simulink model "ES102A_PolarityCfg"
settings: Solver=ode45  StartTime=0.0  StopTime=10.0  RelTol=1e-3
undefined symbols (not defined in the file or in its folder): sigbuilder_block
libraries: simulink x29
(part 2 of 4)

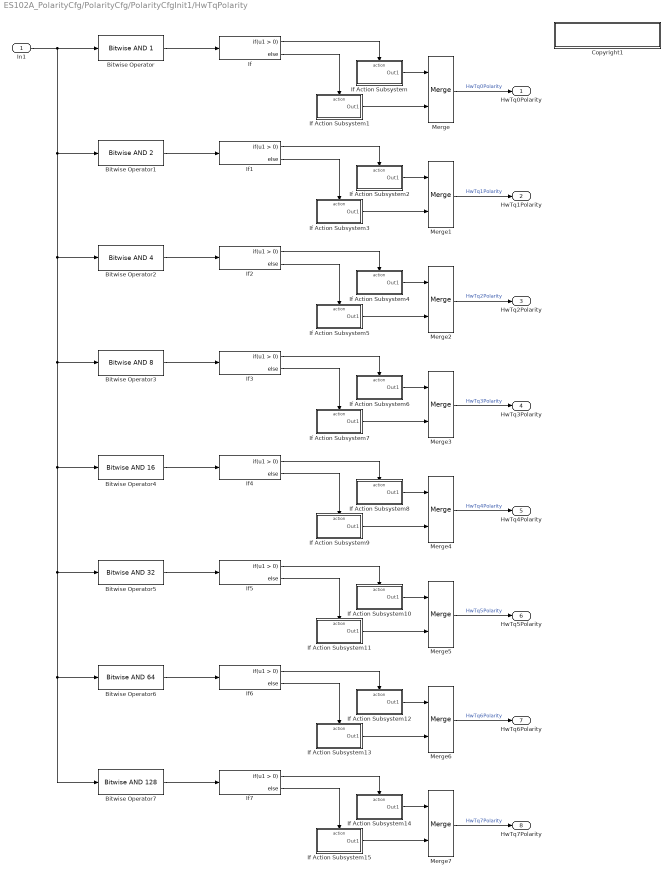
== system ES102A_PolarityCfg/PolarityCfg/PolarityCfgInit1/HwTqPolarity ==
  In1 : Inport
  Bitwise Operator : simulink/Logic and Bit Operations/Bitwise Operator  logicop=AND  UseBitMask=on  BitMask=1  BitMaskRealWorld=Stored Integer
  Bitwise Operator1 : simulink/Logic and Bit Operations/Bitwise Operator  logicop=AND  UseBitMask=on  BitMask=2  BitMaskRealWorld=Stored Integer
  Bitwise Operator2 : simulink/Logic and Bit Operations/Bitwise Operator  logicop=AND  UseBitMask=on  BitMask=4  BitMaskRealWorld=Stored Integer
  Bitwise Operator3 : simulink/Logic and Bit Operations/Bitwise Operator  logicop=AND  UseBitMask=on  BitMask=8  BitMaskRealWorld=Stored Integer
  Bitwise Operator4 : simulink/Logic and Bit Operations/Bitwise Operator  logicop=AND  UseBitMask=on  BitMask=16  BitMaskRealWorld=Stored Integer
  Bitwise Operator5 : simulink/Logic and Bit Operations/Bitwise Operator  logicop=AND  UseBitMask=on  BitMask=32  BitMaskRealWorld=Stored Integer
  Bitwise Operator6 : simulink/Logic and Bit Operations/Bitwise Operator  logicop=AND  UseBitMask=on  BitMask=64  BitMaskRealWorld=Stored Integer
  Bitwise Operator7 : simulink/Logic and Bit Operations/Bitwise Operator  logicop=AND  UseBitMask=on  BitMask=128  BitMaskRealWorld=Stored Integer
  Copyright1 : Subsystem  Description=|  mask(Copyright Information){none=on}
      | Copyright info block.                                               
      |                                                                     
      | Place copyright information at the top of every subsystem in design.
      mask prompts: none "No parameters"
      mask help: Place copyright information at the top of every subsystem in design.
      mask Display:
      | NxtrConf = 'Nexteer Confidential';
      | 
      | sys = bdroot; %handle for the current model ("system")
      | first = get_param(sys,'Created');
      | if(isempty(first))
      |     first = datestr(now,'yyyy');
      | else
      |     first = first(end-3:end);  %year is last four digits
      | end
      | 
      | last = get_param(sys,'LastModifiedDate');
      | if isempty(last)
      |     last = datestr(now,'yyyy');
      | else
      |     last = last(end-3:end);
      | end
      | 
      | if strcmp(first,last)
      |     fprintf('%s\nCopyright  %s Nexteer',NxtrConf,first);
      | else
      |     fprintf('%s\n%s%s-%s Nexteer',NxtrConf,char(169),first,last);
      | end
  If{,1..7} (8 alike) : If
  If Action Subsystem : Subsystem  RequirementInfo={'linktype_rmi_doors' '0000c464 (/ESG Group/FDD Module Requirements/EA4 Specific/ES102A_PolarityCfg_Draft)' '#ES102A_80' 'true' 'REQ: ES102A_80' '' } %GIDa_63d7a222_87e2_4426_b4d4_26a598cfd3d3  TreatAsAtomicUnit=on
  If Action Subsystem1 : Subsystem  RequirementInfo={'linktype_rmi_doors' '0000c464 (/ESG Group/FDD Module Requirements/EA4 Specific/ES102A_PolarityCfg_Draft)' '#ES102A_120' 'true' 'REQ: ES102A_120' '' } %GIDa_21104850_c1b3_421f_933d_f5e3d512e7eb  TreatAsAtomicUnit=on
  If Action Subsystem10 : Subsystem  RequirementInfo={'linktype_rmi_doors' '0000c464 (/ESG Group/FDD Module Requirements/EA4 Specific/ES102A_PolarityCfg_Draft)' '#ES102A_80' 'true' 'REQ: ES102A_80' '' } %GIDa_d3816962_365d_4dbe_9085_fe030921f526  TreatAsAtomicUnit=on
  If Action Subsystem11 : Subsystem  RequirementInfo={'linktype_rmi_doors' '0000c464 (/ESG Group/FDD Module Requirements/EA4 Specific/ES102A_PolarityCfg_Draft)' '#ES102A_120' 'true' 'REQ: ES102A_120' '' } %GIDa_f8f3beb7_25e0_4963_84bd_d008adb7cee4  TreatAsAtomicUnit=on
  If Action Subsystem12 : Subsystem  RequirementInfo={'linktype_rmi_doors' '0000c464 (/ESG Group/FDD Module Requirements/EA4 Specific/ES102A_PolarityCfg_Draft)' '#ES102A_80' 'true' 'REQ: ES102A_80' '' } %GIDa_2ee8a515_44ef_45e2_9975_0d23b295e5d1  TreatAsAtomicUnit=on
  If Action Subsystem13 : Subsystem  RequirementInfo={'linktype_rmi_doors' '0000c464 (/ESG Group/FDD Module Requirements/EA4 Specific/ES102A_PolarityCfg_Draft)' '#ES102A_120' 'true' 'REQ: ES102A_120' '' } %GIDa_ba2a0d96_0e4a_4325_88ca_f247a322979d  TreatAsAtomicUnit=on
  If Action Subsystem14 : Subsystem  RequirementInfo={'linktype_rmi_doors' '0000c464 (/ESG Group/FDD Module Requirements/EA4 Specific/ES102A_PolarityCfg_Draft)' '#ES102A_80' 'true' 'REQ: ES102A_80' '' } %GIDa_1f54eaba_6bb6_4127_a31e_ea55fd3abc1f  TreatAsAtomicUnit=on
  If Action Subsystem15 : Subsystem  RequirementInfo={'linktype_rmi_doors' '0000c464 (/ESG Group/FDD Module Requirements/EA4 Specific/ES102A_PolarityCfg_Draft)' '#ES102A_120' 'true' 'REQ: ES102A_120' '' } %GIDa_c83b58a0_3a0a_4eb5_80bd_66a98f93a285  TreatAsAtomicUnit=on
  If Action Subsystem2 : Subsystem  RequirementInfo={'linktype_rmi_doors' '0000c464 (/ESG Group/FDD Module Requirements/EA4 Specific/ES102A_PolarityCfg_Draft)' '#ES102A_80' 'true' 'REQ: ES102A_80' '' } %GIDa_5262a54c_aaf5_4732_b7ff_1f31c1412e9d  TreatAsAtomicUnit=on
  If Action Subsystem3 : Subsystem  RequirementInfo={'linktype_rmi_doors' '0000c464 (/ESG Group/FDD Module Requirements/EA4 Specific/ES102A_PolarityCfg_Draft)' '#ES102A_120' 'true' 'REQ: ES102A_120' '' } %GIDa_935cd820_58dd_45b1_8f3d_8d9b6ade2195  TreatAsAtomicUnit=on
  If Action Subsystem4 : Subsystem  RequirementInfo={'linktype_rmi_doors' '0000c464 (/ESG Group/FDD Module Requirements/EA4 Specific/ES102A_PolarityCfg_Draft)' '#ES102A_80' 'true' 'REQ: ES102A_80' '' } %GIDa_75b8dd12_95a3_44d6_8e99_0d6e0e3fdd6f  TreatAsAtomicUnit=on
  If Action Subsystem5 : Subsystem  RequirementInfo={'linktype_rmi_doors' '0000c464 (/ESG Group/FDD Module Requirements/EA4 Specific/ES102A_PolarityCfg_Draft)' '#ES102A_120' 'true' 'REQ: ES102A_120' '' } %GIDa_379eacf7_c184_4183_bde5_d58bfea1b961  TreatAsAtomicUnit=on
  If Action Subsystem6 : Subsystem  RequirementInfo={'linktype_rmi_doors' '0000c464 (/ESG Group/FDD Module Requirements/EA4 Specific/ES102A_PolarityCfg_Draft)' '#ES102A_80' 'true' 'REQ: ES102A_80' '' } %GIDa_93f31a74_0cd9_423c_8377_1edcd093e5d6  TreatAsAtomicUnit=on
  If Action Subsystem7 : Subsystem  RequirementInfo={'linktype_rmi_doors' '0000c464 (/ESG Group/FDD Module Requirements/EA4 Specific/ES102A_PolarityCfg_Draft)' '#ES102A_120' 'true' 'REQ: ES102A_120' '' } %GIDa_60e8f548_0e62_4727_b735_42e2eee2da9c  TreatAsAtomicUnit=on
  If Action Subsystem8 : Subsystem  RequirementInfo={'linktype_rmi_doors' '0000c464 (/ESG Group/FDD Module Requirements/EA4 Specific/ES102A_PolarityCfg_Draft)' '#ES102A_80' 'true' 'REQ: ES102A_80' '' } %GIDa_48fc852b_25d9_48ef_8317_b5544d331087  TreatAsAtomicUnit=on
  If Action Subsystem9 : Subsystem  RequirementInfo={'linktype_rmi_doors' '0000c464 (/ESG Group/FDD Module Requirements/EA4 Specific/ES102A_PolarityCfg_Draft)' '#ES102A_120' 'true' 'REQ: ES102A_120' '' } %GIDa_afefc9ee_dd4f_448b_8cdc_7ccd5a68edf1  TreatAsAtomicUnit=on
  Merge : Merge  RequirementInfo={'linktype_rmi_doors' '0000c464 (/ESG Group/FDD Module Requirements/EA4 Specific/ES102A_PolarityCfg_Draft)' '#ES102A_51' 'true' 'REQ: ES102A_51' '' } %GIDa_f47d43ed_cc5a_434e_8d3d_13b3ba273cfe
  Merge1 : Merge  RequirementInfo={'linktype_rmi_doors' '0000c464 (/ESG Group/FDD Module Requirements/EA4 Specific/ES102A_PolarityCfg_Draft)' '#ES102A_96' 'true' 'REQ: ES102A_96' '' } %GIDa_e39f7e38_3c59_4e11_80bf_3cfa32d59145
  Merge2 : Merge  RequirementInfo={'linktype_rmi_doors' '0000c464 (/ESG Group/FDD Module Requirements/EA4 Specific/ES102A_PolarityCfg_Draft)' '#ES102A_97' 'true' 'REQ: ES102A_97' '' } %GIDa_656ea733_9417_4392_8103_592feb91c3e2
  Merge3 : Merge  RequirementInfo={'linktype_rmi_doors' '0000c464 (/ESG Group/FDD Module Requirements/EA4 Specific/ES102A_PolarityCfg_Draft)' '#ES102A_98' 'true' 'REQ: ES102A_98' '' } %GIDa_67ab4764_dfdf_4d10_ad00_44d5b6543dad
  Merge4 : Merge  RequirementInfo={'linktype_rmi_doors' '0000c464 (/ESG Group/FDD Module Requirements/EA4 Specific/ES102A_PolarityCfg_Draft)' '#ES102A_99' 'true' 'REQ: ES102A_99' '' } %GIDa_f01d10c9_6713_4a58_8677_254d13779cb8
  Merge5 : Merge  RequirementInfo={'linktype_rmi_doors' '0000c464 (/ESG Group/FDD Module Requirements/EA4 Specific/ES102A_PolarityCfg_Draft)' '#ES102A_100' 'true' 'REQ: ES102A_100' '' } %GIDa_b89c6608_65de_4443_9860_b993d639af9c
  Merge6 : Merge  RequirementInfo={'linktype_rmi_doors' '0000c464 (/ESG Group/FDD Module Requirements/EA4 Specific/ES102A_PolarityCfg_Draft)' '#ES102A_101' 'true' 'REQ: ES102A_101' '' } %GIDa_62c0d5ff_61a3_4196_82ea_7ef23e77f0bd
  Merge7 : Merge  RequirementInfo={'linktype_rmi_doors' '0000c464 (/ESG Group/FDD Module Requirements/EA4 Specific/ES102A_PolarityCfg_Draft)' '#ES102A_102' 'true' 'REQ: ES102A_102' '' } %GIDa_3c3479f6_5363_44fc_9164_2b7c4fbc1053
  HwTq0Polarity : Outport  RequirementInfo={'doors' '00006113' '48' 'false' 'DOORS Surrogate Item' '' ; 'linktype_rmi_doors' '0000c464 (/ESG Group/FDD Module Requirements/EA4 Specific/ES102A_PolarityCfg_Draft)' '#ES102A_51' 'true' 'REQ: ES102A_51' '' } %GIDa_c470d9f1_1471_4152_8210_a7d10d57422b
  HwTq1Polarity : Outport  RequirementInfo={'doors' '00006113' '49' 'false' 'DOORS Surrogate Item' '' ; 'linktype_rmi_doors' '0000c464 (/ESG Group/FDD Module Requirements/EA4 Specific/ES102A_PolarityCfg_Draft)' '#ES102A_96' 'true' 'REQ: ES102A_96' '' } %GIDa_ed40a89e_763c_4172_ae71_4f4717fd1c6c  Port=2
  HwTq2Polarity : Outport  RequirementInfo={'doors' '00006113' '50' 'false' 'DOORS Surrogate Item' '' ; 'linktype_rmi_doors' '0000c464 (/ESG Group/FDD Module Requirements/EA4 Specific/ES102A_PolarityCfg_Draft)' '#ES102A_97' 'true' 'REQ: ES102A_97' '' } %GIDa_7620c17f_03f2_4abd_85dc_4468565938e3  Port=3
  HwTq3Polarity : Outport  RequirementInfo={'doors' '00006113' '51' 'false' 'DOORS Surrogate Item' '' ; 'linktype_rmi_doors' '0000c464 (/ESG Group/FDD Module Requirements/EA4 Specific/ES102A_PolarityCfg_Draft)' '#ES102A_98' 'true' 'REQ: ES102A_98' '' } %GIDa_eb5c760f_4214_4ac8_9392_ece161eb896a  Port=4
  HwTq4Polarity : Outport  RequirementInfo={'doors' '00006113' '52' 'false' 'DOORS Surrogate Item' '' ; 'linktype_rmi_doors' '0000c464 (/ESG Group/FDD Module Requirements/EA4 Specific/ES102A_PolarityCfg_Draft)' '#ES102A_99' 'true' 'REQ: ES102A_99' '' } %GIDa_111b98a5_5481_44e8_b0fd_d626e710aa2c  Port=5
  HwTq5Polarity : Outport  RequirementInfo={'doors' '00006113' '53' 'false' 'DOORS Surrogate Item' '' ; 'linktype_rmi_doors' '0000c464 (/ESG Group/FDD Module Requirements/EA4 Specific/ES102A_PolarityCfg_Draft)' '#ES102A_100' 'true' 'REQ: ES102A_100' '' } %GIDa_95f59e0f_aa02_4d07_be0c_357d651a5e8c  Port=6
  HwTq6Polarity : Outport  RequirementInfo={'doors' '00006113' '54' 'false' 'DOORS Surrogate Item' '' ; 'linktype_rmi_doors' '0000c464 (/ESG Group/FDD Module Requirements/EA4 Specific/ES102A_PolarityCfg_Draft)' '#ES102A_101' 'true' 'REQ: ES102A_101' '' } %GIDa_e6057f56_db9b_40f9_aef9_186face4720b  Port=7
  HwTq7Polarity : Outport  RequirementInfo={'doors' '00006113' '55' 'false' 'DOORS Surrogate Item' '' ; 'linktype_rmi_doors' '0000c464 (/ESG Group/FDD Module Requirements/EA4 Specific/ES102A_PolarityCfg_Draft)' '#ES102A_102' 'true' 'REQ: ES102A_102' '' } %GIDa_37c293f9_76a2_48d9_8980_8af8f7443fdf  Port=8
  wires:
  Bitwise Operator/1 -> If/1
  If/1 -> If Action Subsystem/Action
  If/2 -> If Action Subsystem1/Action
  If Action Subsystem/1(Out1) -> Merge/1
  If Action Subsystem1/1(Out1) -> Merge/2
  Merge/1 -> HwTq0Polarity/1  "HwTq0Polarity"
  Bitwise Operator1/1 -> If1/1
  If1/1 -> If Action Subsystem2/Action
  If1/2 -> If Action Subsystem3/Action
  If Action Subsystem2/1(Out1) -> Merge1/1
  If Action Subsystem3/1(Out1) -> Merge1/2
  Merge1/1 -> HwTq1Polarity/1  "HwTq1Polarity"
  Bitwise Operator2/1 -> If2/1
  If2/1 -> If Action Subsystem4/Action
  If2/2 -> If Action Subsystem5/Action
  If Action Subsystem4/1(Out1) -> Merge2/1
  If Action Subsystem5/1(Out1) -> Merge2/2
  Merge2/1 -> HwTq2Polarity/1  "HwTq2Polarity"
  Bitwise Operator3/1 -> If3/1
  If3/1 -> If Action Subsystem6/Action
  If3/2 -> If Action Subsystem7/Action
  If Action Subsystem6/1(Out1) -> Merge3/1
  If Action Subsystem7/1(Out1) -> Merge3/2
  Merge3/1 -> HwTq3Polarity/1  "HwTq3Polarity"
  Bitwise Operator4/1 -> If4/1
  If4/1 -> If Action Subsystem8/Action
  If4/2 -> If Action Subsystem9/Action
  If Action Subsystem8/1(Out1) -> Merge4/1
  If Action Subsystem9/1(Out1) -> Merge4/2
  Merge4/1 -> HwTq4Polarity/1  "HwTq4Polarity"
  Bitwise Operator5/1 -> If5/1
  If5/1 -> If Action Subsystem10/Action
  If5/2 -> If Action Subsystem11/Action
  If Action Subsystem10/1(Out1) -> Merge5/1
  If Action Subsystem11/1(Out1) -> Merge5/2
  Merge5/1 -> HwTq5Polarity/1  "HwTq5Polarity"
  In1/1 -> Bitwise Operator2/1, Bitwise Operator7/1, Bitwise Operator6/1, Bitwise Operator5/1, Bitwise Operator4/1, Bitwise Operator3/1, Bitwise Operator1/1, Bitwise Operator/1
  Bitwise Operator6/1 -> If6/1
  If6/1 -> If Action Subsystem12/Action
  If6/2 -> If Action Subsystem13/Action
  If Action Subsystem12/1(Out1) -> Merge6/1
  If Action Subsystem13/1(Out1) -> Merge6/2
  Merge6/1 -> HwTq6Polarity/1  "HwTq6Polarity"
  Bitwise Operator7/1 -> If7/1
  If7/1 -> If Action Subsystem14/Action
  If7/2 -> If Action Subsystem15/Action
  If Action Subsystem14/1(Out1) -> Merge7/1
  If Action Subsystem15/1(Out1) -> Merge7/2
  Merge7/1 -> HwTq7Polarity/1  "HwTq7Polarity"

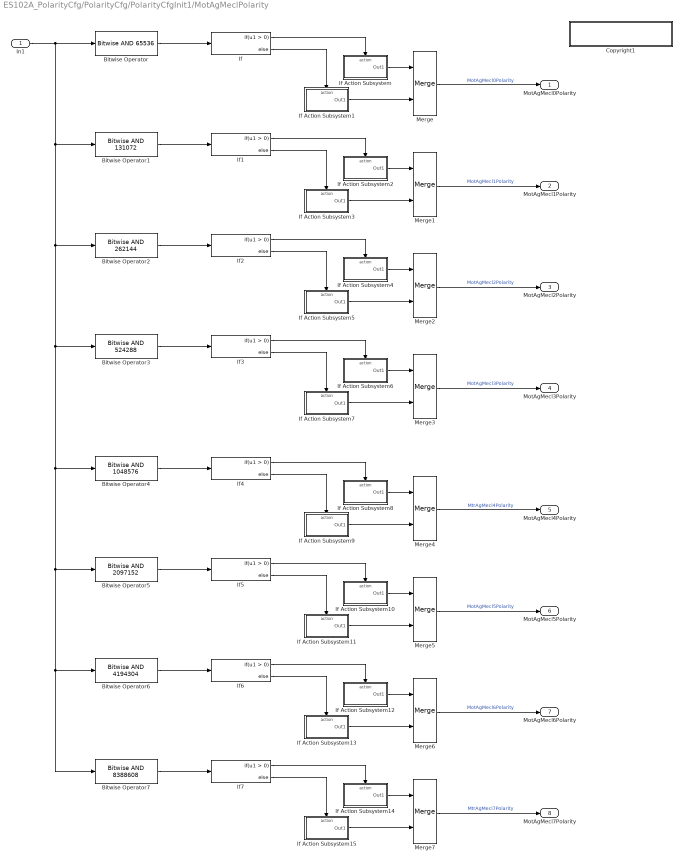
== system ES102A_PolarityCfg/PolarityCfg/PolarityCfgInit1/MotAgMeclPolarity ==
  In1 : Inport
  Bitwise Operator : simulink/Logic and Bit Operations/Bitwise Operator  logicop=AND  UseBitMask=on  BitMask=65536  BitMaskRealWorld=Stored Integer
  Bitwise Operator1 : simulink/Logic and Bit Operations/Bitwise Operator  logicop=AND  UseBitMask=on  BitMask=131072  BitMaskRealWorld=Stored Integer
  Bitwise Operator2 : simulink/Logic and Bit Operations/Bitwise Operator  logicop=AND  UseBitMask=on  BitMask=262144  BitMaskRealWorld=Stored Integer
  Bitwise Operator3 : simulink/Logic and Bit Operations/Bitwise Operator  logicop=AND  UseBitMask=on  BitMask=524288  BitMaskRealWorld=Stored Integer
  Bitwise Operator4 : simulink/Logic and Bit Operations/Bitwise Operator  logicop=AND  UseBitMask=on  BitMask=1048576  BitMaskRealWorld=Stored Integer
  Bitwise Operator5 : simulink/Logic and Bit Operations/Bitwise Operator  logicop=AND  UseBitMask=on  BitMask=2097152  BitMaskRealWorld=Stored Integer
  Bitwise Operator6 : simulink/Logic and Bit Operations/Bitwise Operator  logicop=AND  UseBitMask=on  BitMask=4194304  BitMaskRealWorld=Stored Integer
  Bitwise Operator7 : simulink/Logic and Bit Operations/Bitwise Operator  logicop=AND  UseBitMask=on  BitMask=8388608  BitMaskRealWorld=Stored Integer
  Copyright1 : Subsystem  Description=|  mask(Copyright Information){none=on}
      | Copyright info block.                                               
      |                                                                     
      | Place copyright information at the top of every subsystem in design.
      mask prompts: none "No parameters"
      mask help: Place copyright information at the top of every subsystem in design.
      mask Display:
      | NxtrConf = 'Nexteer Confidential';
      | 
      | sys = bdroot; %handle for the current model ("system")
      | first = get_param(sys,'Created');
      | if(isempty(first))
      |     first = datestr(now,'yyyy');
      | else
      |     first = first(end-3:end);  %year is last four digits
      | end
      | 
      | last = get_param(sys,'LastModifiedDate');
      | if isempty(last)
      |     last = datestr(now,'yyyy');
      | else
      |     last = last(end-3:end);
      | end
      | 
      | if strcmp(first,last)
      |     fprintf('%s\nCopyright  %s Nexteer',NxtrConf,first);
      | else
      |     fprintf('%s\n%s%s-%s Nexteer',NxtrConf,char(169),first,last);
      | end
  If{,1..7} (8 alike) : If
  If Action Subsystem : Subsystem  RequirementInfo={'linktype_rmi_doors' '0000c464 (/ESG Group/FDD Module Requirements/EA4 Specific/ES102A_PolarityCfg_Draft)' '#ES102A_80' 'true' 'REQ: ES102A_80' '' } %GIDa_c5946f2f_0b9f_4812_9390_249c5458628f  TreatAsAtomicUnit=on
  If Action Subsystem1 : Subsystem  RequirementInfo={'linktype_rmi_doors' '0000c464 (/ESG Group/FDD Module Requirements/EA4 Specific/ES102A_PolarityCfg_Draft)' '#ES102A_120' 'true' 'REQ: ES102A_120' '' } %GIDa_17235a92_0b57_4ead_b18c_bc699b71e168  TreatAsAtomicUnit=on
  If Action Subsystem10 : Subsystem  RequirementInfo={'linktype_rmi_doors' '0000c464 (/ESG Group/FDD Module Requirements/EA4 Specific/ES102A_PolarityCfg_Draft)' '#ES102A_80' 'true' 'REQ: ES102A_80' '' } %GIDa_cabfc731_1079_4863_87d4_a2a1f3eed74c  TreatAsAtomicUnit=on
  If Action Subsystem11 : Subsystem  RequirementInfo={'linktype_rmi_doors' '0000c464 (/ESG Group/FDD Module Requirements/EA4 Specific/ES102A_PolarityCfg_Draft)' '#ES102A_120' 'true' 'REQ: ES102A_120' '' } %GIDa_de40052c_f86a_4ed6_a4cf_70244dc4a80a  TreatAsAtomicUnit=on
  If Action Subsystem12 : Subsystem  RequirementInfo={'linktype_rmi_doors' '0000c464 (/ESG Group/FDD Module Requirements/EA4 Specific/ES102A_PolarityCfg_Draft)' '#ES102A_80' 'true' 'REQ: ES102A_80' '' } %GIDa_6ed3d26d_6828_4944_90c2_e0466ba8cbfc  TreatAsAtomicUnit=on
  If Action Subsystem13 : Subsystem  RequirementInfo={'linktype_rmi_doors' '0000c464 (/ESG Group/FDD Module Requirements/EA4 Specific/ES102A_PolarityCfg_Draft)' '#ES102A_120' 'true' 'REQ: ES102A_120' '' } %GIDa_520226fe_c2b8_4250_b652_b1e7aaf239e5  TreatAsAtomicUnit=on
  If Action Subsystem14 : Subsystem  RequirementInfo={'linktype_rmi_doors' '0000c464 (/ESG Group/FDD Module Requirements/EA4 Specific/ES102A_PolarityCfg_Draft)' '#ES102A_80' 'true' 'REQ: ES102A_80' '' } %GIDa_9f63c0d2_98df_422d_9e76_08480bd61c35  TreatAsAtomicUnit=on
  If Action Subsystem15 : Subsystem  RequirementInfo={'linktype_rmi_doors' '0000c464 (/ESG Group/FDD Module Requirements/EA4 Specific/ES102A_PolarityCfg_Draft)' '#ES102A_120' 'true' 'REQ: ES102A_120' '' } %GIDa_c6055289_5356_4833_a678_20f7ef84d772  TreatAsAtomicUnit=on
  If Action Subsystem2 : Subsystem  RequirementInfo={'linktype_rmi_doors' '0000c464 (/ESG Group/FDD Module Requirements/EA4 Specific/ES102A_PolarityCfg_Draft)' '#ES102A_80' 'true' 'REQ: ES102A_80' '' } %GIDa_0192eca6_12f5_480b_91b0_5cfcc8faccb1  TreatAsAtomicUnit=on
  If Action Subsystem3 : Subsystem  RequirementInfo={'linktype_rmi_doors' '0000c464 (/ESG Group/FDD Module Requirements/EA4 Specific/ES102A_PolarityCfg_Draft)' '#ES102A_120' 'true' 'REQ: ES102A_120' '' } %GIDa_d6d5d98a_008b_4639_ba1e_e67d332e29db  TreatAsAtomicUnit=on
  If Action Subsystem4 : Subsystem  RequirementInfo={'linktype_rmi_doors' '0000c464 (/ESG Group/FDD Module Requirements/EA4 Specific/ES102A_PolarityCfg_Draft)' '#ES102A_80' 'true' 'REQ: ES102A_80' '' } %GIDa_3d5fefbf_36ef_4545_87b2_e45a305df674  TreatAsAtomicUnit=on
  If Action Subsystem5 : Subsystem  RequirementInfo={'linktype_rmi_doors' '0000c464 (/ESG Group/FDD Module Requirements/EA4 Specific/ES102A_PolarityCfg_Draft)' '#ES102A_120' 'true' 'REQ: ES102A_120' '' } %GIDa_361beeaf_56ac_433f_8adf_074565dfac65  TreatAsAtomicUnit=on
  If Action Subsystem6 : Subsystem  RequirementInfo={'linktype_rmi_doors' '0000c464 (/ESG Group/FDD Module Requirements/EA4 Specific/ES102A_PolarityCfg_Draft)' '#ES102A_80' 'true' 'REQ: ES102A_80' '' } %GIDa_8efca514_65fe_4817_8fbf_cf5f41ffb619  TreatAsAtomicUnit=on
  If Action Subsystem7 : Subsystem  RequirementInfo={'linktype_rmi_doors' '0000c464 (/ESG Group/FDD Module Requirements/EA4 Specific/ES102A_PolarityCfg_Draft)' '#ES102A_120' 'true' 'REQ: ES102A_120' '' } %GIDa_073176ef_7645_42c7_a94e_900cce625b51  TreatAsAtomicUnit=on
  If Action Subsystem8 : Subsystem  RequirementInfo={'linktype_rmi_doors' '0000c464 (/ESG Group/FDD Module Requirements/EA4 Specific/ES102A_PolarityCfg_Draft)' '#ES102A_80' 'true' 'REQ: ES102A_80' '' } %GIDa_59e259d9_ce1e_4f89_b54a_b64fcb6e78a8  TreatAsAtomicUnit=on
  If Action Subsystem9 : Subsystem  RequirementInfo={'linktype_rmi_doors' '0000c464 (/ESG Group/FDD Module Requirements/EA4 Specific/ES102A_PolarityCfg_Draft)' '#ES102A_120' 'true' 'REQ: ES102A_120' '' } %GIDa_52fcd065_e02d_4289_8673_fa8d1da08e21  TreatAsAtomicUnit=on
  Merge : Merge  RequirementInfo={'linktype_rmi_doors' '0000c464 (/ESG Group/FDD Module Requirements/EA4 Specific/ES102A_PolarityCfg_Draft)' '#ES102A_111' 'true' 'REQ: ES102A_111' '' } %GIDa_1cb9118c_0659_4e90_9a33_0e30e3279ea9
  Merge1 : Merge  RequirementInfo={'linktype_rmi_doors' '0000c464 (/ESG Group/FDD Module Requirements/EA4 Specific/ES102A_PolarityCfg_Draft)' '#ES102A_112' 'true' 'REQ: ES102A_112' '' } %GIDa_01804cea_1b6c_4f32_b834_efb460ab85bd
  Merge2 : Merge  RequirementInfo={'linktype_rmi_doors' '0000c464 (/ESG Group/FDD Module Requirements/EA4 Specific/ES102A_PolarityCfg_Draft)' '#ES102A_113' 'true' 'REQ: ES102A_113' '' } %GIDa_206dd265_0520_4812_b6ee_41059434edda
  Merge3 : Merge  RequirementInfo={'linktype_rmi_doors' '0000c464 (/ESG Group/FDD Module Requirements/EA4 Specific/ES102A_PolarityCfg_Draft)' '#ES102A_114' 'true' 'REQ: ES102A_114' '' } %GIDa_3fafbf9e_b20c_4e77_94f2_328bf7bc39b3
  Merge4 : Merge  RequirementInfo={'linktype_rmi_doors' '0000c464 (/ESG Group/FDD Module Requirements/EA4 Specific/ES102A_PolarityCfg_Draft)' '#ES102A_115' 'true' 'REQ: ES102A_115' '' } %GIDa_7ec066e2_acbd_43a3_b4bc_fc416caebe36
  Merge5 : Merge  RequirementInfo={'linktype_rmi_doors' '0000c464 (/ESG Group/FDD Module Requirements/EA4 Specific/ES102A_PolarityCfg_Draft)' '#ES102A_116' 'true' 'REQ: ES102A_116' '' } %GIDa_e8cb3a86_3d61_44d4_805c_75ed0ab79821
  Merge6 : Merge  RequirementInfo={'linktype_rmi_doors' '0000c464 (/ESG Group/FDD Module Requirements/EA4 Specific/ES102A_PolarityCfg_Draft)' '#ES102A_117' 'true' 'REQ: ES102A_117' '' } %GIDa_625fcab5_94af_4caf_8215_0ddb1120ff87
  Merge7 : Merge  RequirementInfo={'linktype_rmi_doors' '0000c464 (/ESG Group/FDD Module Requirements/EA4 Specific/ES102A_PolarityCfg_Draft)' '#ES102A_118' 'true' 'REQ: ES102A_118' '' } %GIDa_92dfed0d_b9ba_4979_87bf_08f80fe7be37
  MotAgMecl0Polarity : Outport  RequirementInfo={'doors' '00006113' '73' 'false' 'DOORS Surrogate Item' '' ; 'linktype_rmi_doors' '0000c464 (/ESG Group/FDD Module Requirements/EA4 Specific/ES102A_PolarityCfg_Draft)' '#ES102A_111' 'true' 'REQ: ES102A_111' '' } %GIDa_95216d83_d457_4bf2_af30_873833492705
  MotAgMecl1Polarity : Outport  RequirementInfo={'doors' '00006113' '74' 'false' 'DOORS Surrogate Item' '' ; 'linktype_rmi_doors' '0000c464 (/ESG Group/FDD Module Requirements/EA4 Specific/ES102A_PolarityCfg_Draft)' '#ES102A_112' 'true' 'REQ: ES102A_112' '' } %GIDa_ff0e6218_2686_4598_b6b7_fa5f98e64f97  Port=2
  MotAgMecl2Polarity : Outport  RequirementInfo={'doors' '00006113' '75' 'false' 'DOORS Surrogate Item' '' ; 'linktype_rmi_doors' '0000c464 (/ESG Group/FDD Module Requirements/EA4 Specific/ES102A_PolarityCfg_Draft)' '#ES102A_113' 'true' 'REQ: ES102A_113' '' } %GIDa_7394a991_4a99_40ff_9081_355143f46542  Port=3
  MotAgMecl3Polarity : Outport  RequirementInfo={'doors' '00006113' '76' 'false' 'DOORS Surrogate Item' '' ; 'linktype_rmi_doors' '0000c464 (/ESG Group/FDD Module Requirements/EA4 Specific/ES102A_PolarityCfg_Draft)' '#ES102A_114' 'true' 'REQ: ES102A_114' '' } %GIDa_da4aeb3a_9c72_4710_9d7a_5d798e9d90a7  Port=4
  MotAgMecl4Polarity : Outport  RequirementInfo={'doors' '00006113' '77' 'false' 'DOORS Surrogate Item' '' ; 'linktype_rmi_doors' '0000c464 (/ESG Group/FDD Module Requirements/EA4 Specific/ES102A_PolarityCfg_Draft)' '#ES102A_115' 'true' 'REQ: ES102A_115' '' } %GIDa_88a06b38_1492_417e_b5eb_cfb04e1c5553  Port=5
  MotAgMecl5Polarity : Outport  RequirementInfo={'doors' '00006113' '78' 'false' 'DOORS Surrogate Item' '' ; 'linktype_rmi_doors' '0000c464 (/ESG Group/FDD Module Requirements/EA4 Specific/ES102A_PolarityCfg_Draft)' '#ES102A_116' 'true' 'REQ: ES102A_116' '' } %GIDa_e6f50b59_6521_4921_86d4_3e49b0dfffd0  Port=6
  MotAgMecl6Polarity : Outport  RequirementInfo={'doors' '00006113' '79' 'false' 'DOORS Surrogate Item' '' ; 'linktype_rmi_doors' '0000c464 (/ESG Group/FDD Module Requirements/EA4 Specific/ES102A_PolarityCfg_Draft)' '#ES102A_117' 'true' 'REQ: ES102A_117' '' } %GIDa_afa3a81b_308b_4dd4_a88d_b812527054d6  Port=7
  MotAgMecl7Polarity : Outport  RequirementInfo={'doors' '00006113' '80' 'false' 'DOORS Surrogate Item' '' ; 'linktype_rmi_doors' '0000c464 (/ESG Group/FDD Module Requirements/EA4 Specific/ES102A_PolarityCfg_Draft)' '#ES102A_118' 'true' 'REQ: ES102A_118' '' } %GIDa_a990ee8c_3420_4843_8508_80e3dc931edb  Port=8
  wires:
  Bitwise Operator/1 -> If/1
  If/1 -> If Action Subsystem/Action
  If/2 -> If Action Subsystem1/Action
  If Action Subsystem/1(Out1) -> Merge/1
  If Action Subsystem1/1(Out1) -> Merge/2
  Merge/1 -> MotAgMecl0Polarity/1  "MotAgMecl0Polarity"
  Bitwise Operator1/1 -> If1/1
  If1/1 -> If Action Subsystem2/Action
  If1/2 -> If Action Subsystem3/Action
  If Action Subsystem2/1(Out1) -> Merge1/1
  If Action Subsystem3/1(Out1) -> Merge1/2
  Merge1/1 -> MotAgMecl1Polarity/1  "MotAgMecl1Polarity"
  Bitwise Operator2/1 -> If2/1
  If2/1 -> If Action Subsystem4/Action
  If2/2 -> If Action Subsystem5/Action
  If Action Subsystem4/1(Out1) -> Merge2/1
  If Action Subsystem5/1(Out1) -> Merge2/2
  Merge2/1 -> MotAgMecl2Polarity/1  "MotAgMecl2Polarity"
  Bitwise Operator3/1 -> If3/1
  If3/1 -> If Action Subsystem6/Action
  If3/2 -> If Action Subsystem7/Action
  If Action Subsystem6/1(Out1) -> Merge3/1
  If Action Subsystem7/1(Out1) -> Merge3/2
  Merge3/1 -> MotAgMecl3Polarity/1  "MotAgMecl3Polarity"
  Bitwise Operator4/1 -> If4/1
  If4/1 -> If Action Subsystem8/Action
  If4/2 -> If Action Subsystem9/Action
  If Action Subsystem8/1(Out1) -> Merge4/1
  If Action Subsystem9/1(Out1) -> Merge4/2
  Merge4/1 -> MotAgMecl4Polarity/1  "MtrAgMecl4Polarity"
  Bitwise Operator5/1 -> If5/1
  If5/1 -> If Action Subsystem10/Action
  If5/2 -> If Action Subsystem11/Action
  If Action Subsystem10/1(Out1) -> Merge5/1
  If Action Subsystem11/1(Out1) -> Merge5/2
  Merge5/1 -> MotAgMecl5Polarity/1  "MotAgMecl5Polarity"
  In1/1 -> Bitwise Operator2/1, Bitwise Operator6/1, Bitwise Operator7/1, Bitwise Operator5/1, Bitwise Operator4/1, Bitwise Operator3/1, Bitwise Operator1/1, Bitwise Operator/1
  Bitwise Operator6/1 -> If6/1
  If6/1 -> If Action Subsystem12/Action
  If6/2 -> If Action Subsystem13/Action
  If Action Subsystem12/1(Out1) -> Merge6/1
  If Action Subsystem13/1(Out1) -> Merge6/2
  Merge6/1 -> MotAgMecl6Polarity/1  "MotAgMecl6Polarity"
  Bitwise Operator7/1 -> If7/1
  If7/1 -> If Action Subsystem14/Action
  If7/2 -> If Action Subsystem15/Action
  If Action Subsystem14/1(Out1) -> Merge7/1
  If Action Subsystem15/1(Out1) -> Merge7/2
  Merge7/1 -> MotAgMecl7Polarity/1  "MtrAgMecl7Polarity"

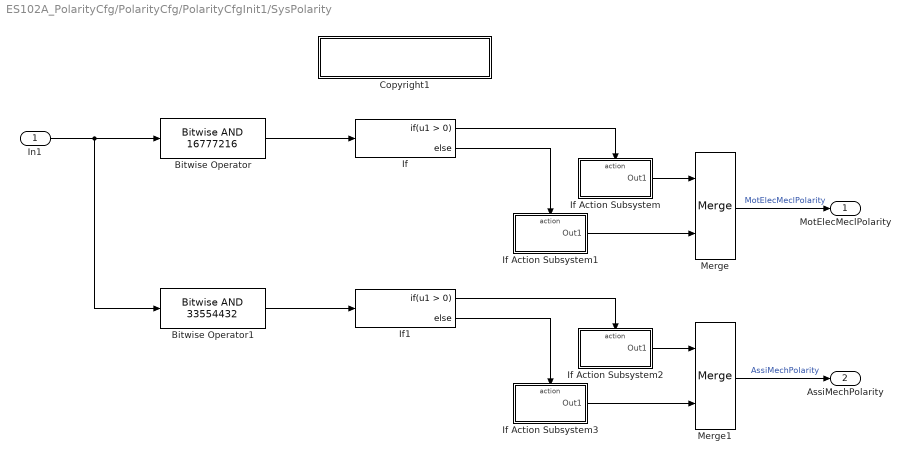
== system ES102A_PolarityCfg/PolarityCfg/PolarityCfgInit1/SysPolarity ==
  In1 : Inport
  Bitwise Operator : simulink/Logic and Bit Operations/Bitwise Operator  logicop=AND  UseBitMask=on  BitMask=16777216  BitMaskRealWorld=Stored Integer
  Bitwise Operator1 : simulink/Logic and Bit Operations/Bitwise Operator  logicop=AND  UseBitMask=on  BitMask=33554432  BitMaskRealWorld=Stored Integer
  Copyright1 : Subsystem  Description=|  mask(Copyright Information){none=on}
      | Copyright info block.                                               
      |                                                                     
      | Place copyright information at the top of every subsystem in design.
      mask prompts: none "No parameters"
      mask help: Place copyright information at the top of every subsystem in design.
      mask Display:
      | NxtrConf = 'Nexteer Confidential';
      | 
      | sys = bdroot; %handle for the current model ("system")
      | first = get_param(sys,'Created');
      | if(isempty(first))
      |     first = datestr(now,'yyyy');
      | else
      |     first = first(end-3:end);  %year is last four digits
      | end
      | 
      | last = get_param(sys,'LastModifiedDate');
      | if isempty(last)
      |     last = datestr(now,'yyyy');
      | else
      |     last = last(end-3:end);
      | end
      | 
      | if strcmp(first,last)
      |     fprintf('%s\nCopyright  %s Nexteer',NxtrConf,first);
      | else
      |     fprintf('%s\n%s%s-%s Nexteer',NxtrConf,char(169),first,last);
      | end
  If : If
  If Action Subsystem : Subsystem  RequirementInfo={'linktype_rmi_doors' '0000c464 (/ESG Group/FDD Module Requirements/EA4 Specific/ES102A_PolarityCfg_Draft)' '#ES102A_80' 'true' 'REQ: ES102A_80' '' } %GIDa_d9e8b945_10d8_4f4e_94d9_8ce26ac6b54b  TreatAsAtomicUnit=on
  If Action Subsystem1 : Subsystem  RequirementInfo={'linktype_rmi_doors' '0000c464 (/ESG Group/FDD Module Requirements/EA4 Specific/ES102A_PolarityCfg_Draft)' '#ES102A_120' 'true' 'REQ: ES102A_120' '' } %GIDa_bc435f67_2244_4529_9754_6b8f8d041ec6  TreatAsAtomicUnit=on
  If Action Subsystem2 : Subsystem  RequirementInfo={'linktype_rmi_doors' '0000c464 (/ESG Group/FDD Module Requirements/EA4 Specific/ES102A_PolarityCfg_Draft)' '#ES102A_80' 'true' 'REQ: ES102A_80' '' } %GIDa_fd742fd1_1f2e_4be3_9489_f2890f4a54eb  TreatAsAtomicUnit=on
  If Action Subsystem3 : Subsystem  RequirementInfo={'linktype_rmi_doors' '0000c464 (/ESG Group/FDD Module Requirements/EA4 Specific/ES102A_PolarityCfg_Draft)' '#ES102A_120' 'true' 'REQ: ES102A_120' '' } %GIDa_84388462_660c_472b_b9a9_b3c4ad928bf4  TreatAsAtomicUnit=on
  If1 : If
  Merge : Merge  RequirementInfo={'linktype_rmi_doors' '0000c464 (/ESG Group/FDD Module Requirements/EA4 Specific/ES102A_PolarityCfg_Draft)' '#ES102A_119' 'true' 'REQ: ES102A_119' '' } %GIDa_42684085_e280_43cc_93a1_7d0e1be79bcf
  Merge1 : Merge  RequirementInfo={'linktype_rmi_doors' '0000c464 (/ESG Group/FDD Module Requirements/EA4 Specific/ES102A_PolarityCfg_Draft)' '#ES102A_124' 'true' 'REQ: ES102A_124' '' } %GIDa_8f3b19c0_6ac2_44b0_9cf3_e074e9794d93
  MotElecMeclPolarity : Outport  RequirementInfo={'doors' '00006113' '98' 'false' 'DOORS Surrogate Item' '' ; 'linktype_rmi_doors' '0000c464 (/ESG Group/FDD Module Requirements/EA4 Specific/ES102A_PolarityCfg_Draft)' '#ES102A_119' 'true' 'REQ: ES102A_119' '' } %GIDa_fc271306_0e1e_4ad7_8e39_60fa997cde00
  AssiMechPolarity : Outport  RequirementInfo={'doors' '00006113' '99' 'false' 'DOORS Surrogate Item' '' ; 'linktype_rmi_doors' '0000c464 (/ESG Group/FDD Module Requirements/EA4 Specific/ES102A_PolarityCfg_Draft)' '#ES102A_124' 'true' 'REQ: ES102A_124' '' } %GIDa_29efb95d_12e9_44c1_aeec_7b34f9c231f1  Port=2
  wires:
  Bitwise Operator/1 -> If/1
  If/1 -> If Action Subsystem/Action
  If/2 -> If Action Subsystem1/Action
  If Action Subsystem/1(Out1) -> Merge/1
  If Action Subsystem1/1(Out1) -> Merge/2
  Merge/1 -> MotElecMeclPolarity/1  "MotElecMeclPolarity"
  Bitwise Operator1/1 -> If1/1
  If1/1 -> If Action Subsystem2/Action
  If1/2 -> If Action Subsystem3/Action
  If Action Subsystem2/1(Out1) -> Merge1/1
  If Action Subsystem3/1(Out1) -> Merge1/2
  Merge1/1 -> AssiMechPolarity/1  "AssiMechPolarity"
  In1/1 -> Bitwise Operator1/1, Bitwise Operator/1

== system ES102A_PolarityCfg/PolarityCfg/PolarityCfgRead/Copyright1 ==

== system ES102A_PolarityCfg/PolarityCfg/PolarityCfgWr/Copyright1 ==

== system ES102A_PolarityCfg/PolarityCfg/PolarityCfgWr/PolarityCfgSaved_SetRamBlockStatus ==
  note: This is the block representing the client call
  BlockChanged : Inport
  Terminator : Terminator
  wires:
  BlockChanged/1 -> Terminator/1

== system ES102A_PolarityCfg/PolarityCfg/PolarityCfgInit1/HwAgPolarity/Copyright1 ==

== system ES102A_PolarityCfg/PolarityCfg/PolarityCfgInit1/HwAgPolarity/If Action Subsystem ==
  Action Port : ActionPort  ActionType=then
  Constant : Constant
  Copyright1 : Subsystem  Description=|  mask(Copyright Information){none=on}
      | Copyright info block.                                               
      |                                                                     
      | Place copyright information at the top of every subsystem in design.
      mask prompts: none "No parameters"
      mask help: Place copyright information at the top of every subsystem in design.
      mask Display:
      | NxtrConf = 'Nexteer Confidential';
      | 
      | sys = bdroot; %handle for the current model ("system")
      | first = get_param(sys,'Created');
      | if(isempty(first))
      |     first = datestr(now,'yyyy');
      | else
      |     first = first(end-3:end);  %year is last four digits
      | end
      | 
      | last = get_param(sys,'LastModifiedDate');
      | if isempty(last)
      |     last = datestr(now,'yyyy');
      | else
      |     last = last(end-3:end);
      | end
      | 
      | if strcmp(first,last)
      |     fprintf('%s\nCopyright  %s Nexteer',NxtrConf,first);
      | else
      |     fprintf('%s\n%s%s-%s Nexteer',NxtrConf,char(169),first,last);
      | end
  Out1 : Outport  InitialOutput=1
  wires:
  Constant/1 -> Out1/1

== system ES102A_PolarityCfg/PolarityCfg/PolarityCfgInit1/HwAgPolarity/If Action Subsystem1 ==
  Action Port : ActionPort  ActionType=else
  Constant : Constant  Value=-1
  Copyright1 : Subsystem  Description=|  mask(Copyright Information){none=on}
      | Copyright info block.                                               
      |                                                                     
      | Place copyright information at the top of every subsystem in design.
      mask prompts: none "No parameters"
      mask help: Place copyright information at the top of every subsystem in design.
      mask Display:
      | NxtrConf = 'Nexteer Confidential';
      | 
      | sys = bdroot; %handle for the current model ("system")
      | first = get_param(sys,'Created');
      | if(isempty(first))
      |     first = datestr(now,'yyyy');
      | else
      |     first = first(end-3:end);  %year is last four digits
      | end
      | 
      | last = get_param(sys,'LastModifiedDate');
      | if isempty(last)
      |     last = datestr(now,'yyyy');
      | else
      |     last = last(end-3:end);
      | end
      | 
      | if strcmp(first,last)
      |     fprintf('%s\nCopyright  %s Nexteer',NxtrConf,first);
      | else
      |     fprintf('%s\n%s%s-%s Nexteer',NxtrConf,char(169),first,last);
      | end
  Out1 : Outport  InitialOutput=-1
  wires:
  Constant/1 -> Out1/1

== system ES102A_PolarityCfg/PolarityCfg/PolarityCfgInit1/HwAgPolarity/If Action Subsystem10 ==
  Action Port : ActionPort  ActionType=then
  Constant : Constant
  Copyright1 : Subsystem  Description=|  mask(Copyright Information){none=on}
      | Copyright info block.                                               
      |                                                                     
      | Place copyright information at the top of every subsystem in design.
      mask prompts: none "No parameters"
      mask help: Place copyright information at the top of every subsystem in design.
      mask Display:
      | NxtrConf = 'Nexteer Confidential';
      | 
      | sys = bdroot; %handle for the current model ("system")
      | first = get_param(sys,'Created');
      | if(isempty(first))
      |     first = datestr(now,'yyyy');
      | else
      |     first = first(end-3:end);  %year is last four digits
      | end
      | 
      | last = get_param(sys,'LastModifiedDate');
      | if isempty(last)
      |     last = datestr(now,'yyyy');
      | else
      |     last = last(end-3:end);
      | end
      | 
      | if strcmp(first,last)
      |     fprintf('%s\nCopyright  %s Nexteer',NxtrConf,first);
      | else
      |     fprintf('%s\n%s%s-%s Nexteer',NxtrConf,char(169),first,last);
      | end
  Out1 : Outport  InitialOutput=1
  wires:
  Constant/1 -> Out1/1

== system ES102A_PolarityCfg/PolarityCfg/PolarityCfgInit1/HwAgPolarity/If Action Subsystem11 ==
  Action Port : ActionPort  ActionType=else
  Constant : Constant  Value=-1
  Copyright1 : Subsystem  Description=|  mask(Copyright Information){none=on}
      | Copyright info block.                                               
      |                                                                     
      | Place copyright information at the top of every subsystem in design.
      mask prompts: none "No parameters"
      mask help: Place copyright information at the top of every subsystem in design.
      mask Display:
      | NxtrConf = 'Nexteer Confidential';
      | 
      | sys = bdroot; %handle for the current model ("system")
      | first = get_param(sys,'Created');
      | if(isempty(first))
      |     first = datestr(now,'yyyy');
      | else
      |     first = first(end-3:end);  %year is last four digits
      | end
      | 
      | last = get_param(sys,'LastModifiedDate');
      | if isempty(last)
      |     last = datestr(now,'yyyy');
      | else
      |     last = last(end-3:end);
      | end
      | 
      | if strcmp(first,last)
      |     fprintf('%s\nCopyright  %s Nexteer',NxtrConf,first);
      | else
      |     fprintf('%s\n%s%s-%s Nexteer',NxtrConf,char(169),first,last);
      | end
  Out1 : Outport  InitialOutput=-1
  wires:
  Constant/1 -> Out1/1

== system ES102A_PolarityCfg/PolarityCfg/PolarityCfgInit1/HwAgPolarity/If Action Subsystem12 ==
  Action Port : ActionPort  ActionType=then
  Constant : Constant
  Copyright1 : Subsystem  Description=|  mask(Copyright Information){none=on}
      | Copyright info block.                                               
      |                                                                     
      | Place copyright information at the top of every subsystem in design.
      mask prompts: none "No parameters"
      mask help: Place copyright information at the top of every subsystem in design.
      mask Display:
      | NxtrConf = 'Nexteer Confidential';
      | 
      | sys = bdroot; %handle for the current model ("system")
      | first = get_param(sys,'Created');
      | if(isempty(first))
      |     first = datestr(now,'yyyy');
      | else
      |     first = first(end-3:end);  %year is last four digits
      | end
      | 
      | last = get_param(sys,'LastModifiedDate');
      | if isempty(last)
      |     last = datestr(now,'yyyy');
      | else
      |     last = last(end-3:end);
      | end
      | 
      | if strcmp(first,last)
      |     fprintf('%s\nCopyright  %s Nexteer',NxtrConf,first);
      | else
      |     fprintf('%s\n%s%s-%s Nexteer',NxtrConf,char(169),first,last);
      | end
  Out1 : Outport  InitialOutput=1
  wires:
  Constant/1 -> Out1/1

== system ES102A_PolarityCfg/PolarityCfg/PolarityCfgInit1/HwAgPolarity/If Action Subsystem13 ==
  Action Port : ActionPort  ActionType=else
  Constant : Constant  Value=-1
  Copyright1 : Subsystem  Description=|  mask(Copyright Information){none=on}
      | Copyright info block.                                               
      |                                                                     
      | Place copyright information at the top of every subsystem in design.
      mask prompts: none "No parameters"
      mask help: Place copyright information at the top of every subsystem in design.
      mask Display:
      | NxtrConf = 'Nexteer Confidential';
      | 
      | sys = bdroot; %handle for the current model ("system")
      | first = get_param(sys,'Created');
      | if(isempty(first))
      |     first = datestr(now,'yyyy');
      | else
      |     first = first(end-3:end);  %year is last four digits
      | end
      | 
      | last = get_param(sys,'LastModifiedDate');
      | if isempty(last)
      |     last = datestr(now,'yyyy');
      | else
      |     last = last(end-3:end);
      | end
      | 
      | if strcmp(first,last)
      |     fprintf('%s\nCopyright  %s Nexteer',NxtrConf,first);
      | else
      |     fprintf('%s\n%s%s-%s Nexteer',NxtrConf,char(169),first,last);
      | end
  Out1 : Outport  InitialOutput=-1
  wires:
  Constant/1 -> Out1/1

== system ES102A_PolarityCfg/PolarityCfg/PolarityCfgInit1/HwAgPolarity/If Action Subsystem14 ==
  Action Port : ActionPort  ActionType=then
  Constant : Constant
  Copyright1 : Subsystem  Description=|  mask(Copyright Information){none=on}
      | Copyright info block.                                               
      |                                                                     
      | Place copyright information at the top of every subsystem in design.
      mask prompts: none "No parameters"
      mask help: Place copyright information at the top of every subsystem in design.
      mask Display:
      | NxtrConf = 'Nexteer Confidential';
      | 
      | sys = bdroot; %handle for the current model ("system")
      | first = get_param(sys,'Created');
      | if(isempty(first))
      |     first = datestr(now,'yyyy');
      | else
      |     first = first(end-3:end);  %year is last four digits
      | end
      | 
      | last = get_param(sys,'LastModifiedDate');
      | if isempty(last)
      |     last = datestr(now,'yyyy');
      | else
      |     last = last(end-3:end);
      | end
      | 
      | if strcmp(first,last)
      |     fprintf('%s\nCopyright  %s Nexteer',NxtrConf,first);
      | else
      |     fprintf('%s\n%s%s-%s Nexteer',NxtrConf,char(169),first,last);
      | end
  Out1 : Outport  InitialOutput=1
  wires:
  Constant/1 -> Out1/1

== system ES102A_PolarityCfg/PolarityCfg/PolarityCfgInit1/HwAgPolarity/If Action Subsystem15 ==
  Action Port : ActionPort  ActionType=else
  Constant : Constant  Value=-1
  Copyright1 : Subsystem  Description=|  mask(Copyright Information){none=on}
      | Copyright info block.                                               
      |                                                                     
      | Place copyright information at the top of every subsystem in design.
      mask prompts: none "No parameters"
      mask help: Place copyright information at the top of every subsystem in design.
      mask Display:
      | NxtrConf = 'Nexteer Confidential';
      | 
      | sys = bdroot; %handle for the current model ("system")
      | first = get_param(sys,'Created');
      | if(isempty(first))
      |     first = datestr(now,'yyyy');
      | else
      |     first = first(end-3:end);  %year is last four digits
      | end
      | 
      | last = get_param(sys,'LastModifiedDate');
      | if isempty(last)
      |     last = datestr(now,'yyyy');
      | else
      |     last = last(end-3:end);
      | end
      | 
      | if strcmp(first,last)
      |     fprintf('%s\nCopyright  %s Nexteer',NxtrConf,first);
      | else
      |     fprintf('%s\n%s%s-%s Nexteer',NxtrConf,char(169),first,last);
      | end
  Out1 : Outport  InitialOutput=-1
  wires:
  Constant/1 -> Out1/1

== system ES102A_PolarityCfg/PolarityCfg/PolarityCfgInit1/HwAgPolarity/If Action Subsystem2 ==
  Action Port : ActionPort  ActionType=then
  Constant : Constant
  Copyright1 : Subsystem  Description=|  mask(Copyright Information){none=on}
      | Copyright info block.                                               
      |                                                                     
      | Place copyright information at the top of every subsystem in design.
      mask prompts: none "No parameters"
      mask help: Place copyright information at the top of every subsystem in design.
      mask Display:
      | NxtrConf = 'Nexteer Confidential';
      | 
      | sys = bdroot; %handle for the current model ("system")
      | first = get_param(sys,'Created');
      | if(isempty(first))
      |     first = datestr(now,'yyyy');
      | else
      |     first = first(end-3:end);  %year is last four digits
      | end
      | 
      | last = get_param(sys,'LastModifiedDate');
      | if isempty(last)
      |     last = datestr(now,'yyyy');
      | else
      |     last = last(end-3:end);
      | end
      | 
      | if strcmp(first,last)
      |     fprintf('%s\nCopyright  %s Nexteer',NxtrConf,first);
      | else
      |     fprintf('%s\n%s%s-%s Nexteer',NxtrConf,char(169),first,last);
      | end
  Out1 : Outport  InitialOutput=1
  wires:
  Constant/1 -> Out1/1

== system ES102A_PolarityCfg/PolarityCfg/PolarityCfgInit1/HwAgPolarity/If Action Subsystem3 ==
  Action Port : ActionPort  ActionType=else
  Constant : Constant  Value=-1
  Copyright1 : Subsystem  Description=|  mask(Copyright Information){none=on}
      | Copyright info block.                                               
      |                                                                     
      | Place copyright information at the top of every subsystem in design.
      mask prompts: none "No parameters"
      mask help: Place copyright information at the top of every subsystem in design.
      mask Display:
      | NxtrConf = 'Nexteer Confidential';
      | 
      | sys = bdroot; %handle for the current model ("system")
      | first = get_param(sys,'Created');
      | if(isempty(first))
      |     first = datestr(now,'yyyy');
      | else
      |     first = first(end-3:end);  %year is last four digits
      | end
      | 
      | last = get_param(sys,'LastModifiedDate');
      | if isempty(last)
      |     last = datestr(now,'yyyy');
      | else
      |     last = last(end-3:end);
      | end
      | 
      | if strcmp(first,last)
      |     fprintf('%s\nCopyright  %s Nexteer',NxtrConf,first);
      | else
      |     fprintf('%s\n%s%s-%s Nexteer',NxtrConf,char(169),first,last);
      | end
  Out1 : Outport  InitialOutput=-1
  wires:
  Constant/1 -> Out1/1

== system ES102A_PolarityCfg/PolarityCfg/PolarityCfgInit1/HwAgPolarity/If Action Subsystem4 ==
  Action Port : ActionPort  ActionType=then
  Constant : Constant
  Copyright1 : Subsystem  Description=|  mask(Copyright Information){none=on}
      | Copyright info block.                                               
      |                                                                     
      | Place copyright information at the top of every subsystem in design.
      mask prompts: none "No parameters"
      mask help: Place copyright information at the top of every subsystem in design.
      mask Display:
      | NxtrConf = 'Nexteer Confidential';
      | 
      | sys = bdroot; %handle for the current model ("system")
      | first = get_param(sys,'Created');
      | if(isempty(first))
      |     first = datestr(now,'yyyy');
      | else
      |     first = first(end-3:end);  %year is last four digits
      | end
      | 
      | last = get_param(sys,'LastModifiedDate');
      | if isempty(last)
      |     last = datestr(now,'yyyy');
      | else
      |     last = last(end-3:end);
      | end
      | 
      | if strcmp(first,last)
      |     fprintf('%s\nCopyright  %s Nexteer',NxtrConf,first);
      | else
      |     fprintf('%s\n%s%s-%s Nexteer',NxtrConf,char(169),first,last);
      | end
  Out1 : Outport  InitialOutput=1
  wires:
  Constant/1 -> Out1/1

== system ES102A_PolarityCfg/PolarityCfg/PolarityCfgInit1/HwAgPolarity/If Action Subsystem5 ==
  Action Port : ActionPort  ActionType=else
  Constant : Constant  Value=-1
  Copyright1 : Subsystem  Description=|  mask(Copyright Information){none=on}
      | Copyright info block.                                               
      |                                                                     
      | Place copyright information at the top of every subsystem in design.
      mask prompts: none "No parameters"
      mask help: Place copyright information at the top of every subsystem in design.
      mask Display:
      | NxtrConf = 'Nexteer Confidential';
      | 
      | sys = bdroot; %handle for the current model ("system")
      | first = get_param(sys,'Created');
      | if(isempty(first))
      |     first = datestr(now,'yyyy');
      | else
      |     first = first(end-3:end);  %year is last four digits
      | end
      | 
      | last = get_param(sys,'LastModifiedDate');
      | if isempty(last)
      |     last = datestr(now,'yyyy');
      | else
      |     last = last(end-3:end);
      | end
      | 
      | if strcmp(first,last)
      |     fprintf('%s\nCopyright  %s Nexteer',NxtrConf,first);
      | else
      |     fprintf('%s\n%s%s-%s Nexteer',NxtrConf,char(169),first,last);
      | end
  Out1 : Outport  InitialOutput=-1
  wires:
  Constant/1 -> Out1/1

== system ES102A_PolarityCfg/PolarityCfg/PolarityCfgInit1/HwAgPolarity/If Action Subsystem6 ==
  Action Port : ActionPort  ActionType=then
  Constant : Constant
  Copyright1 : Subsystem  Description=|  mask(Copyright Information){none=on}
      | Copyright info block.                                               
      |                                                                     
      | Place copyright information at the top of every subsystem in design.
      mask prompts: none "No parameters"
      mask help: Place copyright information at the top of every subsystem in design.
      mask Display:
      | NxtrConf = 'Nexteer Confidential';
      | 
      | sys = bdroot; %handle for the current model ("system")
      | first = get_param(sys,'Created');
      | if(isempty(first))
      |     first = datestr(now,'yyyy');
      | else
      |     first = first(end-3:end);  %year is last four digits
      | end
      | 
      | last = get_param(sys,'LastModifiedDate');
      | if isempty(last)
      |     last = datestr(now,'yyyy');
      | else
      |     last = last(end-3:end);
      | end
      | 
      | if strcmp(first,last)
      |     fprintf('%s\nCopyright  %s Nexteer',NxtrConf,first);
      | else
      |     fprintf('%s\n%s%s-%s Nexteer',NxtrConf,char(169),first,last);
      | end
  Out1 : Outport  InitialOutput=1
  wires:
  Constant/1 -> Out1/1
